simulink model "intelligent_inspection_reference_architecture"  (R2026a)
settings: Solver=VariableStepAuto
Description:
  | Application-independent logical reference architecture. Structural only. Shared workflow version 1.0.0.
settings Model: Creator=Nouran Ismail  LastModifiedBy=Nouran Ismail

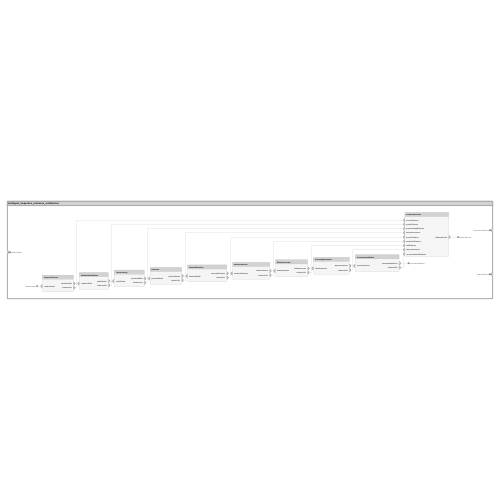
[thumbnail: Simulink's stored preview of the top-level diagram]
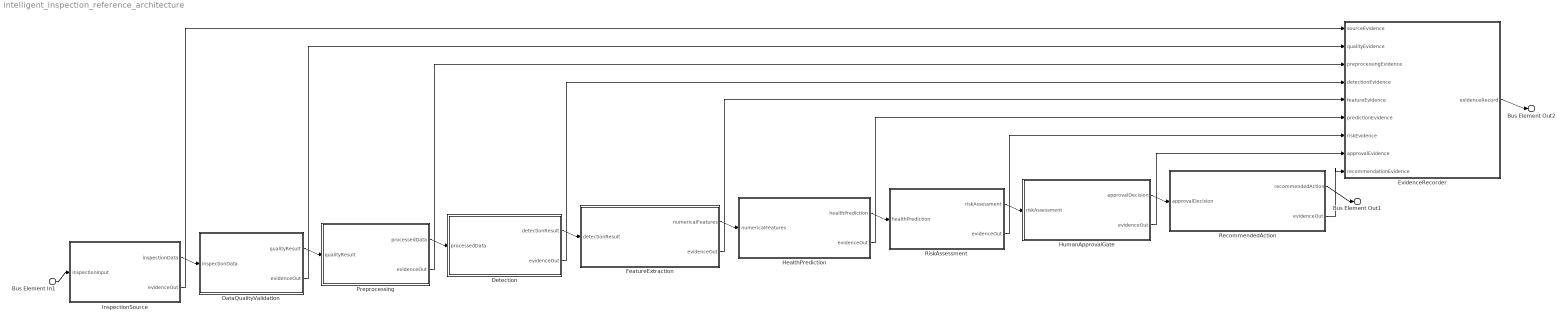
== system intelligent_inspection_reference_architecture ==
  Bus Element In1 : Inport  PortName=inspectionInput
  DataQualityValidation : Subsystem
      settings: PortSchema="{\"entries\":[{\"content\":{\"headerSize\":26,\"margin\":15,\"minimumSpacing\":25,\"sides\":[{\"content\":{\"connectorIds\":[\"In1\"]},\"type\":\"ConnectorPlacement.EquallySpacedRectSide\",\"uuid\":\"3924f80a-bbd7-4543-bdb4-b5bf9ece8fab\"},{\"content\":{\"connectorIds\":[\"Out1\",\"Out2\"],\"side\":\"RIGHT\"},\"type\":\"ConnectorPlacement.EquallySpacedRectSide\",\"uuid\":\"e864e96f-a78e-4353-bb56-fed9dd41a7be\"},{\"content\":{\"side\":\"TOP\"},\"type\":\"ConnectorPlacement.EquallySpacedRectSide\",\"uuid\":\"20f4e367-24be-463a-a956-4711fd391301\"}]},\"type\":\"ConnectorPlacement.EquallySpacedConnector\",\"uuid\":\"e8256b01-81f0-43ff-934b-5a435b3572e2\"}],\"packageUris\":[\"http://schema.mathworks.com/mf0/Connector/R2020b\"],\"version\":\"1.0\"}"
  Detection : Subsystem
      settings: PortSchema="{\"entries\":[{\"content\":{\"headerSize\":26,\"margin\":15,\"minimumSpacing\":25,\"sides\":[{\"content\":{\"connectorIds\":[\"In1\"]},\"type\":\"ConnectorPlacement.EquallySpacedRectSide\",\"uuid\":\"3924f80a-bbd7-4543-bdb4-b5bf9ece8fab\"},{\"content\":{\"connectorIds\":[\"Out1\",\"Out2\"],\"side\":\"RIGHT\"},\"type\":\"ConnectorPlacement.EquallySpacedRectSide\",\"uuid\":\"e864e96f-a78e-4353-bb56-fed9dd41a7be\"},{\"content\":{\"side\":\"TOP\"},\"type\":\"ConnectorPlacement.EquallySpacedRectSide\",\"uuid\":\"20f4e367-24be-463a-a956-4711fd391301\"}]},\"type\":\"ConnectorPlacement.EquallySpacedConnector\",\"uuid\":\"e8256b01-81f0-43ff-934b-5a435b3572e2\"}],\"packageUris\":[\"http://schema.mathworks.com/mf0/Connector/R2020b\"],\"version\":\"1.0\"}"
  EvidenceRecorder : Subsystem
      settings: PortSchema="{\"entries\":[{\"content\":{\"headerSize\":26,\"margin\":15,\"minimumSpacing\":25,\"sides\":[{\"content\":{\"connectorIds\":[\"In1\",\"In2\",\"In3\",\"In4\",\"In5\",\"In6\",\"In7\",\"In8\",\"In9\"]},\"type\":\"ConnectorPlacement.EquallySpacedRectSide\",\"uuid\":\"3924f80a-bbd7-4543-bdb4-b5bf9ece8fab\"},{\"content\":{\"connectorIds\":[\"Out1\"],\"side\":\"RIGHT\"},\"type\":\"ConnectorPlacement.EquallySpacedRectSide\",\"uuid\":\"e864e96f-a78e-4353-bb56-fed9dd41a7be\"},{\"content\":{\"side\":\"TOP\"},\"type\":\"ConnectorPlacement.EquallySpacedRectSide\",\"uuid\":\"20f4e367-24be-463a-a956-4711fd391301\"}]},\"type\":\"ConnectorPlacement.EquallySpacedConnector\",\"uuid\":\"e8256b01-81f0-43ff-934b-5a435b3572e2\"}],\"packageUris\":[\"http://schema.mathworks.com/mf0/Connector/R2020b\"],\"version\":\"1.0\"}"
  FeatureExtraction : Subsystem
      settings: PortSchema="{\"entries\":[{\"content\":{\"headerSize\":26,\"margin\":15,\"minimumSpacing\":25,\"sides\":[{\"content\":{\"connectorIds\":[\"In1\"]},\"type\":\"ConnectorPlacement.EquallySpacedRectSide\",\"uuid\":\"3924f80a-bbd7-4543-bdb4-b5bf9ece8fab\"},{\"content\":{\"connectorIds\":[\"Out1\",\"Out2\"],\"side\":\"RIGHT\"},\"type\":\"ConnectorPlacement.EquallySpacedRectSide\",\"uuid\":\"e864e96f-a78e-4353-bb56-fed9dd41a7be\"},{\"content\":{\"side\":\"TOP\"},\"type\":\"ConnectorPlacement.EquallySpacedRectSide\",\"uuid\":\"20f4e367-24be-463a-a956-4711fd391301\"}]},\"type\":\"ConnectorPlacement.EquallySpacedConnector\",\"uuid\":\"e8256b01-81f0-43ff-934b-5a435b3572e2\"}],\"packageUris\":[\"http://schema.mathworks.com/mf0/Connector/R2020b\"],\"version\":\"1.0\"}"
  HealthPrediction : Subsystem
      settings: PortSchema="{\"entries\":[{\"content\":{\"headerSize\":26,\"margin\":15,\"minimumSpacing\":25,\"sides\":[{\"content\":{\"connectorIds\":[\"In1\"]},\"type\":\"ConnectorPlacement.EquallySpacedRectSide\",\"uuid\":\"3924f80a-bbd7-4543-bdb4-b5bf9ece8fab\"},{\"content\":{\"connectorIds\":[\"Out1\",\"Out2\"],\"side\":\"RIGHT\"},\"type\":\"ConnectorPlacement.EquallySpacedRectSide\",\"uuid\":\"e864e96f-a78e-4353-bb56-fed9dd41a7be\"},{\"content\":{\"side\":\"TOP\"},\"type\":\"ConnectorPlacement.EquallySpacedRectSide\",\"uuid\":\"20f4e367-24be-463a-a956-4711fd391301\"}]},\"type\":\"ConnectorPlacement.EquallySpacedConnector\",\"uuid\":\"e8256b01-81f0-43ff-934b-5a435b3572e2\"}],\"packageUris\":[\"http://schema.mathworks.com/mf0/Connector/R2020b\"],\"version\":\"1.0\"}"
  HumanApprovalGate : Subsystem
      settings: PortSchema="{\"entries\":[{\"content\":{\"headerSize\":26,\"margin\":15,\"minimumSpacing\":25,\"sides\":[{\"content\":{\"connectorIds\":[\"In1\"]},\"type\":\"ConnectorPlacement.EquallySpacedRectSide\",\"uuid\":\"3924f80a-bbd7-4543-bdb4-b5bf9ece8fab\"},{\"content\":{\"connectorIds\":[\"Out1\",\"Out2\"],\"side\":\"RIGHT\"},\"type\":\"ConnectorPlacement.EquallySpacedRectSide\",\"uuid\":\"e864e96f-a78e-4353-bb56-fed9dd41a7be\"},{\"content\":{\"side\":\"TOP\"},\"type\":\"ConnectorPlacement.EquallySpacedRectSide\",\"uuid\":\"20f4e367-24be-463a-a956-4711fd391301\"}]},\"type\":\"ConnectorPlacement.EquallySpacedConnector\",\"uuid\":\"e8256b01-81f0-43ff-934b-5a435b3572e2\"}],\"packageUris\":[\"http://schema.mathworks.com/mf0/Connector/R2020b\"],\"version\":\"1.0\"}"
  InspectionSource : Subsystem
      settings: PortSchema="{\"entries\":[{\"content\":{\"headerSize\":26,\"margin\":15,\"minimumSpacing\":25,\"sides\":[{\"content\":{\"connectorIds\":[\"In1\"]},\"type\":\"ConnectorPlacement.EquallySpacedRectSide\",\"uuid\":\"3924f80a-bbd7-4543-bdb4-b5bf9ece8fab\"},{\"content\":{\"connectorIds\":[\"Out1\",\"Out2\"],\"side\":\"RIGHT\"},\"type\":\"ConnectorPlacement.EquallySpacedRectSide\",\"uuid\":\"e864e96f-a78e-4353-bb56-fed9dd41a7be\"},{\"content\":{\"side\":\"TOP\"},\"type\":\"ConnectorPlacement.EquallySpacedRectSide\",\"uuid\":\"20f4e367-24be-463a-a956-4711fd391301\"}]},\"type\":\"ConnectorPlacement.EquallySpacedConnector\",\"uuid\":\"e8256b01-81f0-43ff-934b-5a435b3572e2\"}],\"packageUris\":[\"http://schema.mathworks.com/mf0/Connector/R2020b\"],\"version\":\"1.0\"}"
  Preprocessing : Subsystem
      settings: PortSchema="{\"entries\":[{\"content\":{\"headerSize\":26,\"margin\":15,\"minimumSpacing\":25,\"sides\":[{\"content\":{\"connectorIds\":[\"In1\"]},\"type\":\"ConnectorPlacement.EquallySpacedRectSide\",\"uuid\":\"3924f80a-bbd7-4543-bdb4-b5bf9ece8fab\"},{\"content\":{\"connectorIds\":[\"Out1\",\"Out2\"],\"side\":\"RIGHT\"},\"type\":\"ConnectorPlacement.EquallySpacedRectSide\",\"uuid\":\"e864e96f-a78e-4353-bb56-fed9dd41a7be\"},{\"content\":{\"side\":\"TOP\"},\"type\":\"ConnectorPlacement.EquallySpacedRectSide\",\"uuid\":\"20f4e367-24be-463a-a956-4711fd391301\"}]},\"type\":\"ConnectorPlacement.EquallySpacedConnector\",\"uuid\":\"e8256b01-81f0-43ff-934b-5a435b3572e2\"}],\"packageUris\":[\"http://schema.mathworks.com/mf0/Connector/R2020b\"],\"version\":\"1.0\"}"
  RecommendedAction : Subsystem
      settings: PortSchema="{\"entries\":[{\"content\":{\"headerSize\":26,\"margin\":15,\"minimumSpacing\":25,\"sides\":[{\"content\":{\"connectorIds\":[\"In1\"]},\"type\":\"ConnectorPlacement.EquallySpacedRectSide\",\"uuid\":\"3924f80a-bbd7-4543-bdb4-b5bf9ece8fab\"},{\"content\":{\"connectorIds\":[\"Out1\",\"Out2\"],\"side\":\"RIGHT\"},\"type\":\"ConnectorPlacement.EquallySpacedRectSide\",\"uuid\":\"e864e96f-a78e-4353-bb56-fed9dd41a7be\"},{\"content\":{\"side\":\"TOP\"},\"type\":\"ConnectorPlacement.EquallySpacedRectSide\",\"uuid\":\"20f4e367-24be-463a-a956-4711fd391301\"}]},\"type\":\"ConnectorPlacement.EquallySpacedConnector\",\"uuid\":\"e8256b01-81f0-43ff-934b-5a435b3572e2\"}],\"packageUris\":[\"http://schema.mathworks.com/mf0/Connector/R2020b\"],\"version\":\"1.0\"}"
  RiskAssessment : Subsystem
      settings: PortSchema="{\"entries\":[{\"content\":{\"headerSize\":26,\"margin\":15,\"minimumSpacing\":25,\"sides\":[{\"content\":{\"connectorIds\":[\"In1\"]},\"type\":\"ConnectorPlacement.EquallySpacedRectSide\",\"uuid\":\"3924f80a-bbd7-4543-bdb4-b5bf9ece8fab\"},{\"content\":{\"connectorIds\":[\"Out1\",\"Out2\"],\"side\":\"RIGHT\"},\"type\":\"ConnectorPlacement.EquallySpacedRectSide\",\"uuid\":\"e864e96f-a78e-4353-bb56-fed9dd41a7be\"},{\"content\":{\"side\":\"TOP\"},\"type\":\"ConnectorPlacement.EquallySpacedRectSide\",\"uuid\":\"20f4e367-24be-463a-a956-4711fd391301\"}]},\"type\":\"ConnectorPlacement.EquallySpacedConnector\",\"uuid\":\"e8256b01-81f0-43ff-934b-5a435b3572e2\"}],\"packageUris\":[\"http://schema.mathworks.com/mf0/Connector/R2020b\"],\"version\":\"1.0\"}"
  Bus Element Out1 : Outport  PortName=recommendedAction
  Bus Element Out2 : Outport  Port=2  PortName=evidenceRecord
  wires:
  Preprocessing/2(evidenceOut) -> EvidenceRecorder/3(preprocessingEvidence)
  Preprocessing/1(processedData) -> Detection/1(processedData)
  Bus Element In1/1 -> InspectionSource/1(inspectionInput)
  InspectionSource/2(evidenceOut) -> EvidenceRecorder/1(sourceEvidence)
  RecommendedAction/1(recommendedAction) -> Bus Element Out1/1
  InspectionSource/1(inspectionData) -> DataQualityValidation/1(inspectionData)
  DataQualityValidation/2(evidenceOut) -> EvidenceRecorder/2(qualityEvidence)
  DataQualityValidation/1(qualityResult) -> Preprocessing/1(qualityResult)
  Detection/1(detectionResult) -> FeatureExtraction/1(detectionResult)
  Detection/2(evidenceOut) -> EvidenceRecorder/4(detectionEvidence)
  FeatureExtraction/1(numericalFeatures) -> HealthPrediction/1(numericalFeatures)
  FeatureExtraction/2(evidenceOut) -> EvidenceRecorder/5(featureEvidence)
  HealthPrediction/1(healthPrediction) -> RiskAssessment/1(healthPrediction)
  HealthPrediction/2(evidenceOut) -> EvidenceRecorder/6(predictionEvidence)
  RiskAssessment/1(riskAssessment) -> HumanApprovalGate/1(riskAssessment)
  RiskAssessment/2(evidenceOut) -> EvidenceRecorder/7(riskEvidence)
  HumanApprovalGate/1(approvalDecision) -> RecommendedAction/1(approvalDecision)
  HumanApprovalGate/2(evidenceOut) -> EvidenceRecorder/8(approvalEvidence)
  RecommendedAction/2(evidenceOut) -> EvidenceRecorder/9(recommendationEvidence)
  EvidenceRecorder/1(evidenceRecord) -> Bus Element Out2/1

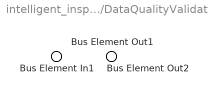
== system intelligent_inspection_reference_architecture/DataQualityValidation ==
  Bus Element In1 : Inport  PortName=inspectionData
  Bus Element Out1 : Outport  PortName=qualityResult
  Bus Element Out2 : Outport  Port=2  PortName=evidenceOut

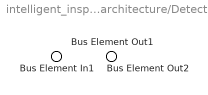
== system intelligent_inspection_reference_architecture/Detection ==
  Bus Element In1 : Inport  PortName=processedData
  Bus Element Out1 : Outport  PortName=detectionResult
  Bus Element Out2 : Outport  Port=2  PortName=evidenceOut

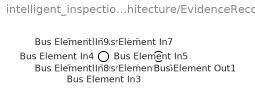
== system intelligent_inspection_reference_architecture/EvidenceRecorder ==
  Bus Element In1 : Inport  PortName=sourceEvidence
  Bus Element In2 : Inport  Port=2  PortName=qualityEvidence
  Bus Element In3 : Inport  Port=3  PortName=preprocessingEvidence
  Bus Element In4 : Inport  Port=4  PortName=detectionEvidence
  Bus Element In5 : Inport  Port=5  PortName=featureEvidence
  Bus Element In6 : Inport  Port=6  PortName=predictionEvidence
  Bus Element In7 : Inport  Port=7  PortName=riskEvidence
  Bus Element In8 : Inport  Port=8  PortName=approvalEvidence
  Bus Element In9 : Inport  Port=9  PortName=recommendationEvidence
  Bus Element Out1 : Outport  PortName=evidenceRecord

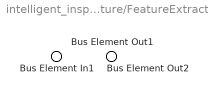
== system intelligent_inspection_reference_architecture/FeatureExtraction ==
  Bus Element In1 : Inport  PortName=detectionResult
  Bus Element Out1 : Outport  PortName=numericalFeatures
  Bus Element Out2 : Outport  Port=2  PortName=evidenceOut

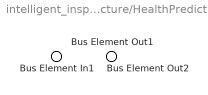
== system intelligent_inspection_reference_architecture/HealthPrediction ==
  Bus Element In1 : Inport  PortName=numericalFeatures
  Bus Element Out1 : Outport  PortName=healthPrediction
  Bus Element Out2 : Outport  Port=2  PortName=evidenceOut

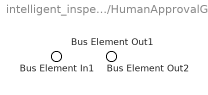
== system intelligent_inspection_reference_architecture/HumanApprovalGate ==
  Bus Element In1 : Inport  PortName=riskAssessment
  Bus Element Out1 : Outport  PortName=approvalDecision
  Bus Element Out2 : Outport  Port=2  PortName=evidenceOut

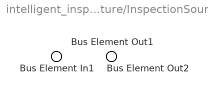
== system intelligent_inspection_reference_architecture/InspectionSource ==
  Bus Element In1 : Inport  PortName=inspectionInput
  Bus Element Out1 : Outport  PortName=inspectionData
  Bus Element Out2 : Outport  Port=2  PortName=evidenceOut

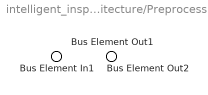
== system intelligent_inspection_reference_architecture/Preprocessing ==
  Bus Element In1 : Inport  PortName=qualityResult
  Bus Element Out1 : Outport  PortName=processedData
  Bus Element Out2 : Outport  Port=2  PortName=evidenceOut

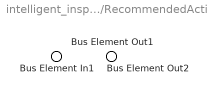
== system intelligent_inspection_reference_architecture/RecommendedAction ==
  Bus Element In1 : Inport  PortName=approvalDecision
  Bus Element Out1 : Outport  PortName=recommendedAction
  Bus Element Out2 : Outport  Port=2  PortName=evidenceOut

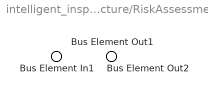
== system intelligent_inspection_reference_architecture/RiskAssessment ==
  Bus Element In1 : Inport  PortName=healthPrediction
  Bus Element Out1 : Outport  PortName=riskAssessment
  Bus Element Out2 : Outport  Port=2  PortName=evidenceOut
